simulink model "WaterRunner_ground"  (Simulink 7.9)
settings: Solver=ode15s  StartTime=0.0  StopTime=5  RelTol=1e-6
InitFcn:
  | simParams
StartFcn:
  | simParams
undefined symbols (not defined in the file or in its folder): water_level
libraries: WaterRunner_lib x17, mblibv1 x4, simulink x1
settings Model: Creator=fumiyaiida  LastModifiedBy=nitisht  SimulationMode=accelerator
settings SolverCC: ZeroCrossControl=DisableAll  SolverResetMethod=Robust
settings OptimizationCC: InlineInvariantSignals=on  InitFltsAndDblsToZero=on  EfficientMapNaN2IntZero=off  SimCompilerOptimization=On
settings DebuggingCC: SaveWithParameterizedLinksMsg=none  SignalResolutionControl=TryResolveAllWithWarning  MultiTaskDSMMsg=warning  MultiTaskCondExecSysMsg=none  FcnCallInpInsideContextMsg=Use local settings  StrictBusMsg=None
settings HardwareCC: ProdBitPerLong=64  ProdBitPerPointer=64  ProdIntDivRoundTo=Zero  ProdEndianess=LittleEndian  ProdWordSize=64  ProdHWDeviceType=Intel->x86-64  TargetBitPerLong=64  TargetBitPerPointer=64  TargetIntDivRoundTo=Zero  TargetEndianess=LittleEndian  TargetWordSize=64  TargetHWDeviceType=MATLAB Host  ProdEqTarget=off
settings CodeAppCC: MaxIdLength=128
settings GRTTargetCC: CombineOutputUpdateFcns=off  GRTInterface=on
settings SimMechanicsCC: WarnOnSingularInitialAssembly=on  VisOnUpdateDiagram=on  VisDuringSimulation=on  VisSampleTime=0.008  AnimationDelay=1  LastVizWinPosition=[2 461 1918 517]  CamPosition=[1.00064;2.69855;15.1508;]  CamTarget=[2.34303;0.595283;-0.252842;]  CamUpVector=[-0.0141613;0.990541;-0.136486;]  CamHeight=1.71731  VisBackgroundColor=[0.9;0.9;0.95;]  DefaultBodyColor=[1;0;0;]  MDLBodyVisualizationType=Equivalent ellipsoid from mass properties
settings ConfigurationSet: Description=SimMechanics 2G

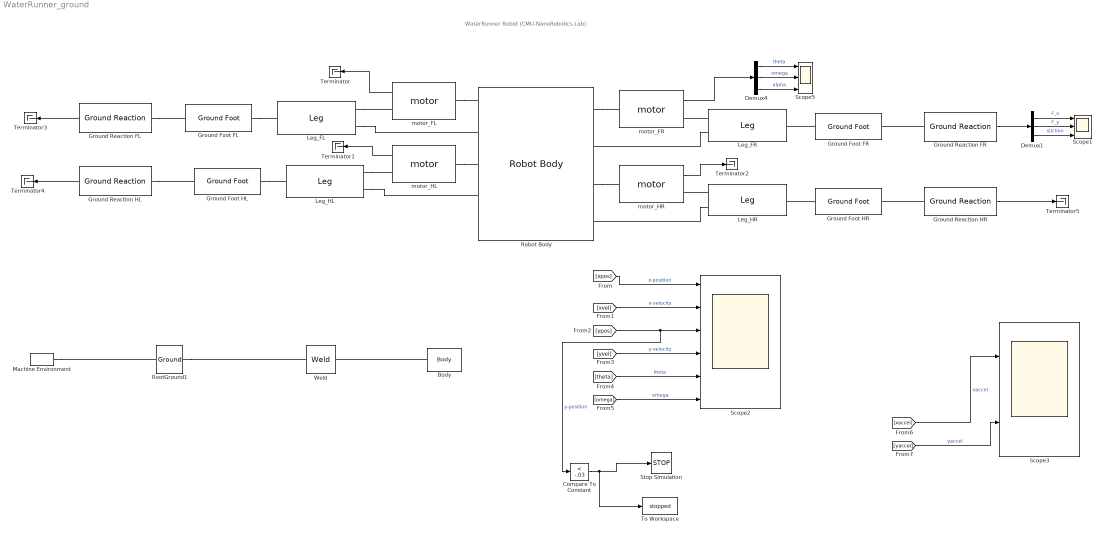
== system WaterRunner_ground ==
  note: WaterRunner Robot
      | (CMU-NanoRobotics Lab)
  Body : mblibv1/Bodies/Body  LConnTagsString=CG  UpdateFromCAD=off  DialogClass=MechanicalBodyBlock  Mass=1  MassUnits=kg  InertiaUnits=kg*m^2  Inertia=eye(3)  Shape=Cylinder  ShapeDims=[1 1]  ShapeUnits=m  ShapeUse=false  Density=1  DensityUnits=kg/m^3  DensityUse=false  GraphicsMode=CONVHULL  BodyColorSelMode=COLORPALETTE  BodyColor=[0.83137 0.81569 0.78431]  AttachedToCS=CG  CG=Left$CG$[0 0 0]$WORLD$WORLD$m$[0 0 0]$Euler X-Y-Z$deg$WORLD$true$none  WorkingFrames=Left$CS1$[-0.5 water_level -0.2 ]$CG$CG$m$[0 0 0]$Euler X-Y-Z$deg$WORLD$false$none#Left$CS2$[-0.5 water_level 0.2 ]$CG$CG$m$[0 0 0]$Euler X-Y-Z$deg$WORLD$false$none#Left$CS3$[4 water_level -0.2 ]$CG$CG$m$[0 0 0]$Euler X-Y-Z$deg$WORLD$false$none#Left$CS4$[4 water_level 0.2 ]$CG$CG$m$[0 0 0]$Euler X-Y-Z$deg$WORLD$false$none  CGPos=[0 0 0]  CGRot=[0 0 0]  CS0Pos=[]  CS0Rot=[]  CS1Pos=[-0.5 water_level -0.2 ]  CS1Rot=[0 0 0]  CS2Pos=[-0.5 water_level 0.2 ]  CS2Rot=[0 0 0]  CS3Pos=[4 water_level -0.2 ]  CS3Rot=[0 0 0]  CS4Pos=[4 water_level 0.2 ]  CS4Rot=[0 0 0]  CS5Pos=[]  CS5Rot=[]  CS6Pos=[]  CS6Rot=[]  CS7Pos=[]  CS7Rot=[]  CS8Pos=[]  CS8Rot=[]  CS9Pos=[]  CS9Rot=[]  CS10Pos=[]  CS10Rot=[]  CS11Pos=[]  CS11Rot=[]  CS12Pos=[]  CS12Rot=[]  CS13Pos=[]  CS13Rot=[]  CS14Pos=[]  CS14Rot=[]  CS15Pos=[]  CS15Rot=[]  CS16Pos=[]  CS16Rot=[]  CS17Pos=[]  CS17Rot=[]  CS18Pos=[]  CS18Rot=[]  CS19Pos=[]  CS19Rot=[]  CS20Pos=[]  CS20Rot=[]
  Compare To Constant : simulink/Logic and Bit Operations/Compare To Constant  relop=<  const=-.03  OutDataTypeStr=boolean
  Demux1 : Demux  Outputs=3
  Demux4 : Demux  Outputs=3
  Ground Foot FL : WaterRunner_lib/Ground Foot
  Ground Foot FR : WaterRunner_lib/Ground Foot
  Ground Foot HL : WaterRunner_lib/Ground Foot
  Ground Foot HR : WaterRunner_lib/Ground Foot
  Ground Reaction FL : WaterRunner_lib/Ground Reaction
  Ground Reaction FR : WaterRunner_lib/Ground Reaction
  Ground Reaction HL : WaterRunner_lib/Ground Reaction
  Ground Reaction HR : WaterRunner_lib/Ground Reaction
  Leg_FL : WaterRunner_lib/Leg
  Leg_FR : WaterRunner_lib/Leg
  Leg_HL : WaterRunner_lib/Leg
  Leg_HR : WaterRunner_lib/Leg
  Machine Environment : mblibv1/Bodies/Machine Environment  PortType=env  PhysicalDomain=Mechanical  DialogTemplateClass=MECH.MachineEnvironment  SyncWhenCopied=off  Gravity=[0 -9.81 0]  GravityUnits=m/s^2  GravityAsSignal=off  Dimensionality=Auto-detect  AnalysisType=Forward dynamics  LinearAssemblyTolerance=1e-3  LinearAssemblyToleranceUnits=m  AngularAssemblyTolerance=1e-3  AngularAssemblyToleranceUnits=rad  ConstraintSolverType=Stabilizing  ConstraintRelTolerance=1e-4  ConstraintAbsTolerance=1e-4  UseRobustSingularityHandling=off  RedundancyAnalysisToleranceType=Automatically select tolerance  RedundancyAnalysisTolerance=1e-14  StatePerturbationType=Fixed  PerturbationSize=1e-5  VisualizeMachine=on  BodyVisualizationType=Use model default body geometries  BodyColorSelMode=Use model default  DefaultBodyColor=[1 0 0]
  Robot Body : WaterRunner_lib/Robot Body  initRobHeight=initRobHeight
  RootGround1 : mblibv1/Bodies/Ground  UpdateFromCAD=on  LeftPortType=env  RightPortType=workingframe  PhysicalDomain=Mechanical  DialogClass=GroundBlock  CoordPosition=[0 0 0]  CoordPositionUnits=m  StateVectorMgrId=3  MachineId=[2 0]  ShowEnvPort=on
  Scope1 : Scope  NumInputPorts=3
      settings: TimeRange=2  YMin=-1250~0~-70000  YMax=500~1500~30000  SaveName=footForce
  Scope2 : Scope  NumInputPorts=6
      settings: ShowLegends=on  TimeRange=2  YMin=0~0~-1.38778e-17~-1.5~-0.1~-7.5  YMax=2~3.5~0.2~1.5~0.8~10  SaveName=position
  Scope3 : Scope  NumInputPorts=2
      settings: ShowLegends=on  TimeRange=2  YMin=-15~-17.5  YMax=22.5~30  SaveName=position1
  Scope5 : Scope  NumInputPorts=3
      settings: TimeRange=2  YMin=-17.5~-90~-70000  YMax=0~0~30000  SaveName=MotorMotion
  Stop Simulation : Stop
  Terminator{,1..5} (6 alike) : Terminator
  To Workspace : ToWorkspace  VariableName=stopped  SampleTime=-1  SaveFormat=Timeseries
  Weld : mblibv1/Joints/Weld  LConnTagsString=__newl0  RConnTagsString=__newr0  UpdateFromCAD=off  NumSAPorts=0  CutJoint=off  MarkAsCut=off  Primitives=weld  PrimitiveProps=W$WORLD$[0 0 0]$weld  DialogClass=JointBlock  WAxis=[0 0 0]
  motor_FL : WaterRunner_lib/motor  variableName=work_FL  ic_angle=pi
  motor_FR : WaterRunner_lib/motor  variableName=work_FR  ic_angle=0
  motor_HL : WaterRunner_lib/motor  variableName=work_HL  ic_angle=0
  motor_HR : WaterRunner_lib/motor  variableName=work_HR  ic_angle=pi
  wires:
  [xpos] -> Scope2/1  "x-position"
  [xvel] -> Scope2/2  "x-velocity"
  [ypos] -> Scope2/3, Compare To Constant/1  "y-position"
  [yvel] -> Scope2/4  "y-velocity"
  [omega] -> Scope2/6  "omega"
  [theta] -> Scope2/5  "theta"
  Compare To Constant/1 -> Stop Simulation/1, To Workspace/1
  Demux4/3 -> Scope5/3  "alpha"
  Demux4/2 -> Scope5/2  "omega"
  Demux4/1 -> Scope5/1  "theta"
  motor_FR/1 -> Demux4/1
  motor_FL/1 -> Terminator/1
  motor_HL/1 -> Terminator1/1
  motor_HR/1 -> Terminator2/1
  Demux1/3 -> Scope1/3  "stiction"
  Demux1/2 -> Scope1/2  "F_y"
  Demux1/1 -> Scope1/1  "F_x"
  Ground Reaction FR/1 -> Demux1/1
  Ground Reaction FL/1 -> Terminator3/1
  Ground Reaction HL/1 -> Terminator4/1
  Ground Reaction HR/1 -> Terminator5/1
  [xaccel] -> Scope3/1  "xaccel"
  [yaccel] -> Scope3/2  "yaccel"
  connections:
  Robot Body/RConn1 -- motor_FR/LConn1
  Leg_FR/LConn2 -- Robot Body/RConn2
  Leg_FR/LConn1 -- motor_FR/RConn1
  Body/LConn1 -- Weld/RConn1
  RootGround1/RConn1 -- Weld/LConn1
  Machine Environment/RConn1 -- RootGround1/LConn1
  Ground Foot FR/LConn1 -- Leg_FR/RConn1
  Leg_HR/LConn2 -- Robot Body/RConn4
  Leg_HR/LConn1 -- motor_HR/RConn1
  Ground Foot HR/LConn1 -- Leg_HR/RConn1
  Robot Body/RConn3 -- motor_HR/LConn1
  motor_FL/LConn1 -- Robot Body/LConn1
  Leg_FL/LConn1 -- motor_FL/RConn1
  Leg_FL/LConn2 -- Robot Body/LConn2
  Ground Foot FL/LConn1 -- Leg_FL/RConn1
  Leg_HL/LConn1 -- motor_HL/RConn1
  motor_HL/LConn1 -- Robot Body/LConn3
  Ground Foot HL/LConn1 -- Leg_HL/RConn1
  Leg_HL/LConn2 -- Robot Body/LConn4
  Ground Reaction HR/LConn1 -- Ground Foot HR/RConn1
  Ground Reaction FR/LConn1 -- Ground Foot FR/RConn1
  Ground Reaction FL/LConn1 -- Ground Foot FL/RConn1
  Ground Reaction HL/LConn1 -- Ground Foot HL/RConn1
